simulink model "PendSwingUp"  (Simulink 8.6)
settings: Solver=ode1  SolverMode=SingleTasking  StartTime=0.0  StopTime=40  FixedStep=0.001  RelTol=1e-3
undefined symbols (not defined in the file): Advantech, PCI
libraries: sldrtlib x11, simulink x2
settings Model: Creator=pawel  LastModifiedBy=demo  SimulationMode=external  ExtModeTrigMode=oneshot  ExtModeTrigDuration=100000
settings DataIOCC: LimitDataPoints=off  SignalLoggingName=sigsOut
settings OptimizationCC: BlockReduction=off  BooleanDataType=off  InitFltsAndDblsToZero=on
settings DebuggingCC: SaveWithParameterizedLinksMsg=none  SignalResolutionControl=TryResolveAllWithWarning  SolverPrmCheckMsg=none  MultiTaskDSMMsg=warning  MultiTaskCondExecSysMsg=none  FcnCallInpInsideContextMsg=UseLocalSettings
settings HardwareCC: ProdBitPerLong=64  ProdBitPerPointer=64  ProdIntDivRoundTo=Zero  ProdEndianess=LittleEndian  ProdWordSize=64  ProdHWDeviceType=Intel->x86-64  TargetBitPerLong=64  TargetBitPerPointer=64  TargetIntDivRoundTo=Zero  TargetEndianess=LittleEndian  TargetWordSize=64  TargetHWDeviceType=Intel->x86-64
settings RTWCC: SystemTargetFile=sldrt.tlc  TemplateMakefile=sldrt.tmf  Description=Simulink Desktop Real-Time  RTWCompilerOptimization=on
settings CodeAppCC: MaxIdLength=95
settings SimulinkDesktopRealTimeCC: TargetPreCompLibLocation=C:\Program Files\MATLAB\R2015b\toolbox\sldrt\lib\win64  TargetLangStandard=C89/C90 (ANSI)  SupportVariableSizeSignals=off

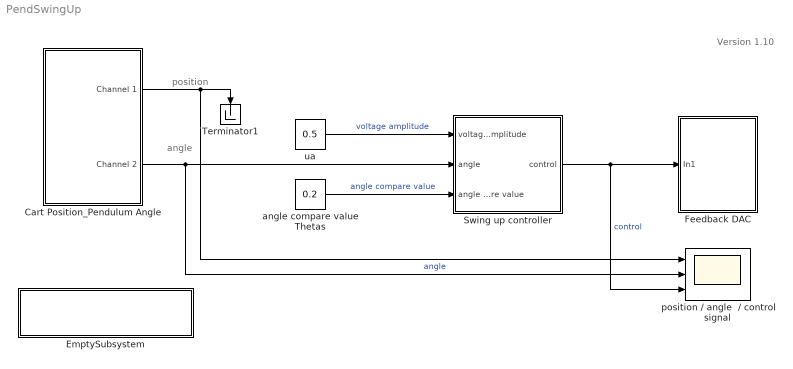
== system PendSwingUp ==
  note: position
  note: angle
  note: Version 1.10
  Cart Position_Pendulum Angle : Subsystem  mask(Feedback Encoder Block){st=0.001, of1=0, of2=-1024}
      mask prompts: st "Sample Time"; of1 "Channel 1 Offset"; of2 "Channel 2 Offset"
      mask help: Special block to use with the Feedback experiments to read encoder channels using the digital I/O lines
      mask Display:
      | image(imread('bckg.bmp'))
      | disp('PCI1711 \n Lab I/O Board \n\n\n Feedback Encoder')
  EmptySubsystem : Subsystem
      mask Display:
      | image(imread('FB-inst-blue2.jpg'))
      | disp('\n\nFeedback Instruments Limited')
  Feedback DAC : Subsystem  mask(DAC Unit for Feedback Experiments){st=0.001, ch=1}
      mask prompts: st "Sample Time"; ch "Output Channel"
      mask help:
      | Digital to Analog Output  for Feedback Experiments
      | using Advantech PCI1711  I/O board
      mask Display:
      | image(imread('bckg.bmp'))
      | disp('PCI1711 \n Lab I/O Board \n\n Feedback  DAC')
  Swing up controller : Subsystem
      mask Display:
      | image(imread('bckg.bmp'))
      | disp('Swing up \ncontroller')
  Terminator1 : Terminator
  angle compare value Thetas : Constant  Value=0.2
  position / angle  / control signal : Scope  NumInputPorts=3
      mask Display: image(imread('scope.jpg'))
  ua : Constant  Value=0.5
  wires:
  ua/1 -> Swing up controller/1(voltage amplitude)  "voltage amplitude"
  angle compare value Thetas/1 -> Swing up controller/3(angle compare value)  "angle compare value"
  Swing up controller/1(control) -> Feedback DAC/1(In1), position / angle  / control signal/3  "control"
  Cart Position_Pendulum Angle/1(Channel 1) -> Terminator1/1, position / angle  / control signal/1
  Cart Position_Pendulum Angle/2(Channel 2) -> Swing up controller/2(angle), position / angle  / control signal/2  "angle"

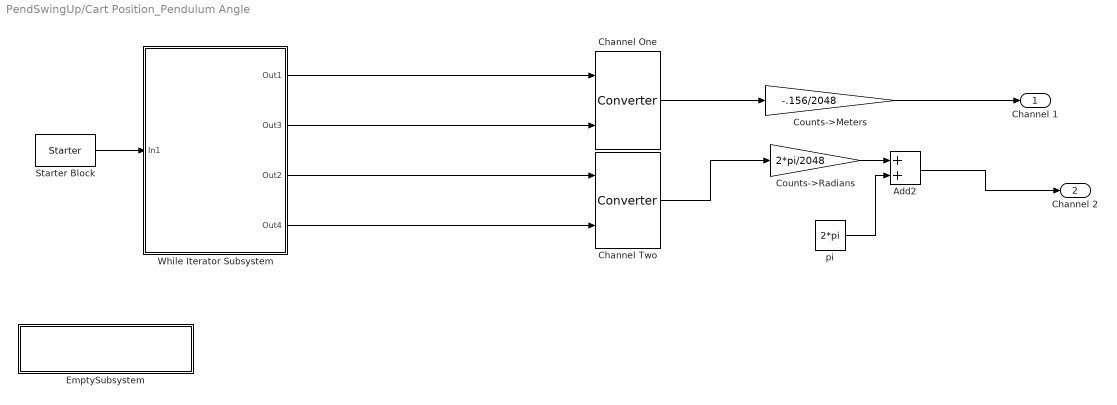
== system PendSwingUp/Cart Position_Pendulum Angle ==
  Add2 : Sum
  Channel One : S-Function  FunctionName=Converter  Parameters=of1,st  SFunctionDeploymentMode=off  EnableBusSupport=off
  Channel Two : S-Function  FunctionName=Converter  Parameters=of2,st  SFunctionDeploymentMode=off  EnableBusSupport=off
  Counts->Meters : Gain  Gain=-.156/2048  SaturateOnIntegerOverflow=on  OutDataTypeStr=Inherit: Same as input  ParamDataTypeStr=Inherit: Same as input
  Counts->Radians : Gain  Gain=2*pi/2048  SaturateOnIntegerOverflow=on  OutDataTypeStr=Inherit: Same as input  ParamDataTypeStr=Inherit: Same as input
  EmptySubsystem : Subsystem
      mask Display:
      | image(imread('FB-inst-blue2.jpg'))
      | disp('\n\nFeedback Instruments Limited')
  Starter Block : S-Function  FunctionName=Starter  Parameters=sample_time  SFunctionDeploymentMode=off  EnableBusSupport=off  mask{sample_time=st}
      mask prompts: sample_time "Sample Time:"
  While Iterator Subsystem : Subsystem  TreatAsAtomicUnit=on
  pi : Constant  Value=2*pi
  Channel 1 : Outport
  Channel 2 : Outport  Port=2
  wires:
  Add2/1 -> Channel 2/1
  Channel Two/1 -> Counts->Radians/1
  pi/1 -> Add2/2
  Counts->Radians/1 -> Add2/1
  Counts->Meters/1 -> Channel 1/1
  Starter Block/1 -> While Iterator Subsystem/1(In1)
  While Iterator Subsystem/1(Out1) -> Channel One/1
  While Iterator Subsystem/2(Out3) -> Channel One/2
  While Iterator Subsystem/3(Out2) -> Channel Two/1
  While Iterator Subsystem/4(Out4) -> Channel Two/2
  Channel One/1 -> Counts->Meters/1

== system PendSwingUp/EmptySubsystem ==

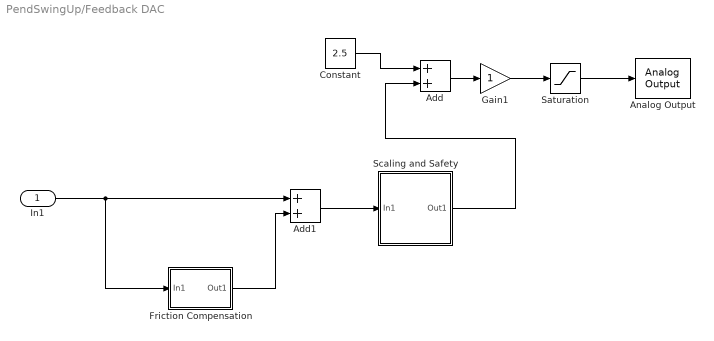
== system PendSwingUp/Feedback DAC ==
  In1 : Inport
  Add : Sum  OutDataTypeStr=Inherit: Same as first input
  Add1 : Sum
  Analog Output : sldrtlib/Analog Output  SampleTime=st  MaxMissedTicks=10  ShowMissedTicks=off  YieldWhenWaiting=off  DrvName=Advantech/PCI-1711  DrvAddress=4294967295  DrvOptions=zeros(1,0)  Channels=ch  RangeMode=1  VoltRange=2  InitialValue=2.5  FinalValue=2.5
      settings: AttributesFormatString=Advantech\nPCI-1711 [auto]
  Constant : Constant  Value=2.5
  Friction Compensation : Subsystem  mask(linear){frictionCompNeg=.1, frictionCompPos=.1}
      mask prompts: frictionCompNeg "Friction Compensation Magnitude in Negative Direction"; frictionCompPos "Friction Compensation Magnitude in Positive Direction"
      mask Display: plot(0,0,100,100,[40,30,20],[87,85,80],[46,54,54,46,46],[90,90,80,80,90],[46,45,45,46,54,55,55,54,46],[78,80,90,91,91,90,80,78,78],[51,51,49,49],[78,10,10,78],[90,80,70,60],[70,80,85,88],[20,10],[80,70],[20,20,15],[73,80,80],[85,80,80],[80,80,74])
  Gain1 : Gain
  Saturation : Saturate  UpperLimit=5.0  LowerLimit=0
  Scaling and Safety : Subsystem
  wires:
  Add1/1 -> Scaling and Safety/1(In1)
  In1/1 -> Add1/1, Friction Compensation/1(In1)
  Friction Compensation/1(Out1) -> Add1/2
  Constant/1 -> Add/1
  Saturation/1 -> Analog Output/1
  Add/1 -> Gain1/1
  Gain1/1 -> Saturation/1
  Scaling and Safety/1(Out1) -> Add/2

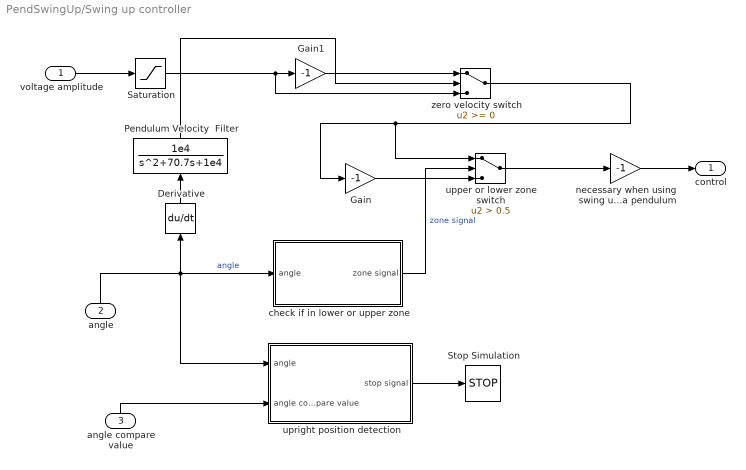
== system PendSwingUp/Swing up controller ==
  voltage amplitude : Inport
  angle : Inport  Port=2
  angle compare value : Inport  Port=3
  Derivative : Derivative
  Gain : Gain  Gain=-1
  Gain1 : Gain  Gain=-1
  Pendulum Velocity  Filter : TransferFcn  Numerator=[1e4]  Denominator=[1 70.7 1e4]
  Saturation : Saturate  UpperLimit=1  LowerLimit=0.01
  Stop Simulation : Stop
  check if in lower or upper zone : Subsystem
      mask Display:
      | image(imread('bckg.bmp'))
      | disp('lower / upper zone')
  necessary when using  swing up on a pendulum : Gain  Gain=-1
  upper or lower zone switch : Switch  Criteria=u2 > Threshold  Threshold=0.5
  upright position detection : Subsystem
      mask Display:
      | image(imread('bckg.bmp'))
      | disp('Upright position \ndetection')
  zero velocity switch : Switch
  control : Outport
  wires:
  angle compare value/1 -> upright position detection/2(angle compare value)
  angle/1 -> upright position detection/1(angle), check if in lower or upper zone/1(angle), Derivative/1  "angle"
  upright position detection/1(stop signal) -> Stop Simulation/1
  upper or lower zone switch/1 -> necessary when using  swing up on a pendulum/1
  zero velocity switch/1 -> upper or lower zone switch/1, Gain/1
  Gain1/1 -> zero velocity switch/1
  voltage amplitude/1 -> Saturation/1
  Gain/1 -> upper or lower zone switch/3
  check if in lower or upper zone/1(zone signal) -> upper or lower zone switch/2  "zone signal"
  Derivative/1 -> Pendulum Velocity  Filter/1
  Pendulum Velocity  Filter/1 -> zero velocity switch/2
  necessary when using  swing up on a pendulum/1 -> control/1
  Saturation/1 -> Gain1/1, zero velocity switch/3

== system PendSwingUp/Cart Position_Pendulum Angle/EmptySubsystem ==

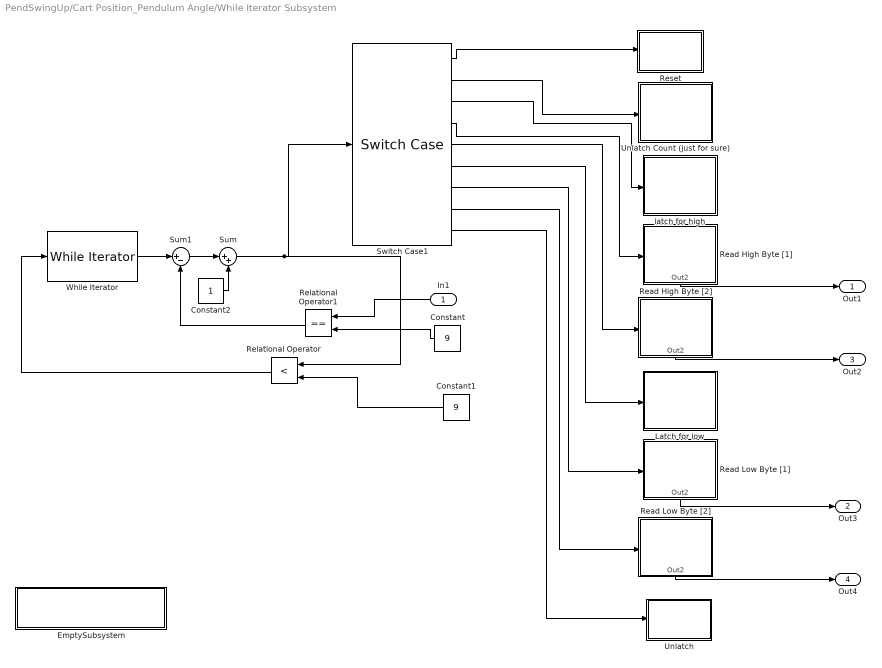
== system PendSwingUp/Cart Position_Pendulum Angle/While Iterator Subsystem ==
  In1 : Inport
  Constant : Constant  Value=9
  Constant1 : Constant  Value=9
  Constant2 : Constant
  EmptySubsystem : Subsystem
      mask Display:
      | image(imread('FB-inst-blue2.jpg'))
      | disp('\n\nFeedback Instruments Limited')
  Latch for low : Subsystem  TreatAsAtomicUnit=on
  Read High Byte [1] : Subsystem  TreatAsAtomicUnit=on
  Read High Byte [2] : Subsystem  TreatAsAtomicUnit=on
  Read Low Byte [1] : Subsystem  TreatAsAtomicUnit=on
  Read Low Byte [2] : Subsystem  TreatAsAtomicUnit=on
  Relational Operator : RelationalOperator  Operator=<  OutDataTypeStr=boolean
  Relational Operator1 : RelationalOperator  Operator===  OutDataTypeStr=boolean
  Reset : Subsystem  TreatAsAtomicUnit=on
  Sum : Sum  Inputs=|++
  Sum1 : Sum  Inputs=|+-  OutDataTypeStr=Inherit: Same as first input
  Switch Case1 : SwitchCase  CaseConditions={1,2,3,4,5,6,7,8,9}  ShowDefaultCase=off
  Unlatch : Subsystem  TreatAsAtomicUnit=on
  "Unlatch Count (just for sure) " : Subsystem  TreatAsAtomicUnit=on
  While Iterator : WhileIterator  MaxIters=9  WhileBlockType=do-while  ResetStates=reset  ShowIterationPort=on  OutputDataType=int8
  latch for high : Subsystem  TreatAsAtomicUnit=on
  Out1 : Outport
  Out3 : Outport  Port=2
  Out2 : Outport  Port=3
  Out4 : Outport  Port=4
  wires:
  Relational Operator/1 -> While Iterator/1
  In1/1 -> Relational Operator1/1
  Constant/1 -> Relational Operator1/2
  Relational Operator1/1 -> Sum1/2
  While Iterator/1 -> Sum1/1
  Switch Case1/1 -> Reset/Action
  Switch Case1/2 -> "Unlatch Count (just for sure) "/Action
  Constant1/1 -> Relational Operator/2
  Read High Byte [1]/1(Out2) -> Out1/1
  Read High Byte [2]/1(Out2) -> Out2/1
  Read Low Byte [1]/1(Out2) -> Out3/1
  Read Low Byte [2]/1(Out2) -> Out4/1
  Sum1/1 -> Sum/1
  Sum/1 -> Switch Case1/1, Relational Operator/1
  Constant2/1 -> Sum/2
  Switch Case1/3 -> latch for high/Action
  Switch Case1/4 -> Read High Byte [1]/Action
  Switch Case1/5 -> Read High Byte [2]/Action
  Switch Case1/6 -> Latch for low/Action
  Switch Case1/7 -> Read Low Byte [1]/Action
  Switch Case1/8 -> Read Low Byte [2]/Action
  Switch Case1/9 -> Unlatch/Action

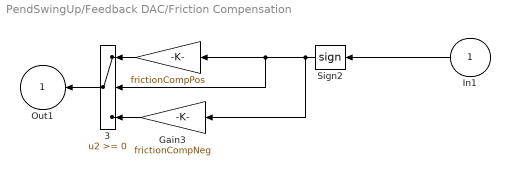
== system PendSwingUp/Feedback DAC/Friction Compensation ==
  In1 : Inport
  " " : Gain  Gain=frictionCompPos  SaturateOnIntegerOverflow=on  OutDataTypeStr=Inherit: Same as input  ParamDataTypeStr=Inherit: Same as input
  3 : Switch  SaturateOnIntegerOverflow=on  InputSameDT=on
  Gain3 : Gain  Gain=frictionCompNeg  SaturateOnIntegerOverflow=on  OutDataTypeStr=Inherit: Same as input  ParamDataTypeStr=Inherit: Same as input
  Sign2 : Signum  Tag=T
  Out1 : Outport  InitialOutput=0
  wires:
  3/1 -> Out1/1
  Sign2/1 -> 3/2, " "/1, Gain3/1
  Gain3/1 -> 3/3
  " "/1 -> 3/1
  In1/1 -> Sign2/1

== system PendSwingUp/Feedback DAC/Scaling and Safety ==
  In1 : Inport
  -1 : Gain  Gain=-1  SaturateOnIntegerOverflow=on  OutDataTypeStr=Inherit: Same as input  ParamDataTypeStr=Inherit: Same as input
  Saturation : Saturate  UpperLimit=2.5  LowerLimit=-2.5
  Out1 : Outport
  wires:
  -1/1 -> Saturation/1  "actual LoadPosition"
  In1/1 -> -1/1
  Saturation/1 -> Out1/1

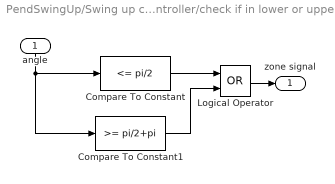
== system PendSwingUp/Swing up controller/check if in lower or upper zone ==
  angle : Inport
  Compare To Constant : simulink/Logic and Bit Operations/Compare To Constant  relop=<=  const=pi/2  OutDataTypeStr=uint8  ZeroCross=off
  Compare To Constant1 : simulink/Logic and Bit Operations/Compare To Constant  relop=>=  const=pi/2+pi  OutDataTypeStr=uint8  ZeroCross=off
  Logical Operator : Logic  Operator=OR  AllPortsSameDT=off  OutDataTypeStr=boolean
  zone signal : Outport
  wires:
  Logical Operator/1 -> zone signal/1
  angle/1 -> Compare To Constant1/1, Compare To Constant/1
  Compare To Constant1/1 -> Logical Operator/2
  Compare To Constant/1 -> Logical Operator/1

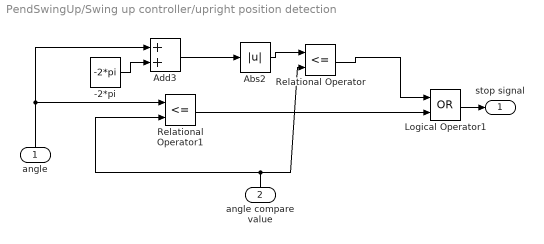
== system PendSwingUp/Swing up controller/upright position detection ==
  angle : Inport
  angle compare value : Inport  Port=2
  -2*pi : Constant  Value=-2*pi
  Abs2 : Abs
  Add3 : Sum
  Logical Operator1 : Logic  Operator=OR  AllPortsSameDT=off  OutDataTypeStr=boolean
  Relational Operator : RelationalOperator  Operator=<=  OutDataTypeStr=boolean
  Relational Operator1 : RelationalOperator  Operator=<=  OutDataTypeStr=boolean
  stop signal : Outport
  wires:
  angle compare value/1 -> Relational Operator1/2, Relational Operator/2
  Logical Operator1/1 -> stop signal/1
  angle/1 -> Relational Operator1/1, Add3/1
  Abs2/1 -> Relational Operator/1
  Add3/1 -> Abs2/1
  Relational Operator/1 -> Logical Operator1/1
  -2*pi/1 -> Add3/2
  Relational Operator1/1 -> Logical Operator1/2

== system PendSwingUp/Cart Position_Pendulum Angle/While Iterator Subsystem/EmptySubsystem ==

== system PendSwingUp/Cart Position_Pendulum Angle/While Iterator Subsystem/Latch for low ==
  Action Port : ActionPort  ActionType=case
  Constant : Constant  Value=6  OutDataTypeStr=double
  Digital Output : sldrtlib/Digital Output  SampleTime=-1  MaxMissedTicks=10  ShowMissedTicks=off  YieldWhenWaiting=off  DrvName=Advantech/PCI-1711  DrvAddress=4294967295  DrvOptions=zeros(1,0)  Channels=1  BitMode=2  InitialValue=0  FinalValue=0
      settings: AttributesFormatString=Advantech\nPCI-1711 [auto]
  wires:
  Constant/1 -> Digital Output/1

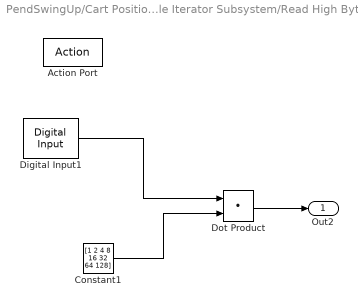
== system PendSwingUp/Cart Position_Pendulum Angle/While Iterator Subsystem/Read High Byte [1] ==
  Action Port : ActionPort  ActionType=case
  Constant1 : Constant  Value=[1 2 4 8 16 32 64 128]
  Digital Input1 : sldrtlib/Digital Input  SampleTime=-1  MaxMissedTicks=10  ShowMissedTicks=off  YieldWhenWaiting=off  DrvName=Advantech/PCI-1711  DrvAddress=4294967295  DrvOptions=zeros(1,0)  Channels=[1,2,3,4,5,6,7,8]  BitMode=1  DataType=1
      settings: AttributesFormatString=Advantech\nPCI-1711 [auto]
  Dot Product : DotProduct  InputSameDT=on  OutDataTypeStr=Inherit: Inherit via internal rule
  Out2 : Outport
  wires:
  Dot Product/1 -> Out2/1
  Constant1/1 -> Dot Product/2
  Digital Input1/1 -> Dot Product/1

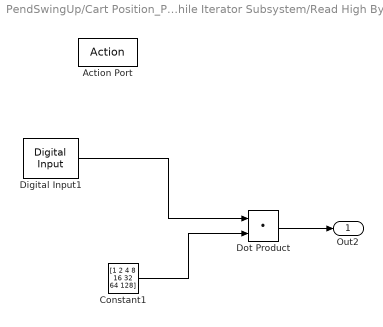
== system PendSwingUp/Cart Position_Pendulum Angle/While Iterator Subsystem/Read High Byte [2] ==
  Action Port : ActionPort  ActionType=case
  Constant1 : Constant  Value=[1 2 4 8 16 32 64 128]
  Digital Input1 : sldrtlib/Digital Input  SampleTime=-1  MaxMissedTicks=10  ShowMissedTicks=off  YieldWhenWaiting=off  DrvName=Advantech/PCI-1711  DrvAddress=4294967295  DrvOptions=zeros(1,0)  Channels=[9:16]  BitMode=1  DataType=1
      settings: AttributesFormatString=Advantech\nPCI-1711 [auto]
  Dot Product : DotProduct  InputSameDT=on  OutDataTypeStr=Inherit: Inherit via internal rule
  Out2 : Outport
  wires:
  Digital Input1/1 -> Dot Product/1
  Constant1/1 -> Dot Product/2
  Dot Product/1 -> Out2/1

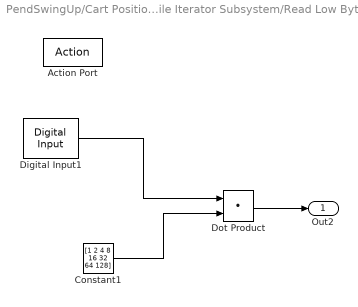
== system PendSwingUp/Cart Position_Pendulum Angle/While Iterator Subsystem/Read Low Byte [1] ==
  Action Port : ActionPort  ActionType=case
  Constant1 : Constant  Value=[1 2 4 8 16 32 64 128]
  Digital Input1 : sldrtlib/Digital Input  SampleTime=-1  MaxMissedTicks=10  ShowMissedTicks=off  YieldWhenWaiting=off  DrvName=Advantech/PCI-1711  DrvAddress=4294967295  DrvOptions=zeros(1,0)  Channels=[1:8]  BitMode=1  DataType=1
      settings: AttributesFormatString=Advantech\nPCI-1711 [auto]
  Dot Product : DotProduct  InputSameDT=on  OutDataTypeStr=Inherit: Inherit via internal rule
  Out2 : Outport
  wires:
  Digital Input1/1 -> Dot Product/1
  Constant1/1 -> Dot Product/2
  Dot Product/1 -> Out2/1

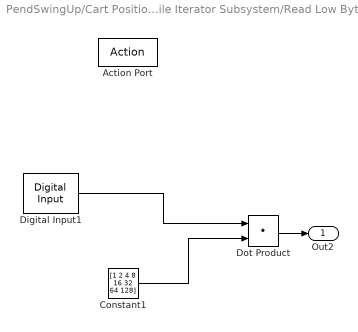
== system PendSwingUp/Cart Position_Pendulum Angle/While Iterator Subsystem/Read Low Byte [2] ==
  Action Port : ActionPort  ActionType=case
  Constant1 : Constant  Value=[1 2 4 8 16 32 64 128]
  Digital Input1 : sldrtlib/Digital Input  SampleTime=-1  MaxMissedTicks=10  ShowMissedTicks=off  YieldWhenWaiting=off  DrvName=Advantech/PCI-1711  DrvAddress=4294967295  DrvOptions=zeros(1,0)  Channels=[9:16]  BitMode=1  DataType=1
      settings: AttributesFormatString=Advantech\nPCI-1711 [auto]
  Dot Product : DotProduct  InputSameDT=on  OutDataTypeStr=Inherit: Inherit via internal rule
  Out2 : Outport
  wires:
  Constant1/1 -> Dot Product/2
  Digital Input1/1 -> Dot Product/1
  Dot Product/1 -> Out2/1

== system PendSwingUp/Cart Position_Pendulum Angle/While Iterator Subsystem/Reset ==
  Action Port : ActionPort  ActionType=case
  Constant : Constant  Value=3  OutDataTypeStr=double
  Digital Output1 : sldrtlib/Digital Output  SampleTime=-1  MaxMissedTicks=10  ShowMissedTicks=off  YieldWhenWaiting=off  DrvName=Advantech/PCI-1711  DrvAddress=4294967295  DrvOptions=zeros(1,0)  Channels=1  BitMode=2  InitialValue=0  FinalValue=0
      settings: AttributesFormatString=Advantech\nPCI-1711 [auto]
  Subsystem : Subsystem
  wires:
  Constant/1 -> Subsystem/1(In1)
  Subsystem/1(Out1) -> Digital Output1/1

== system PendSwingUp/Cart Position_Pendulum Angle/While Iterator Subsystem/Unlatch ==
  Action Port : ActionPort  ActionType=case
  Constant : Constant  Value=7  OutDataTypeStr=double
  Digital Output1 : sldrtlib/Digital Output  SampleTime=-1  MaxMissedTicks=10  ShowMissedTicks=off  YieldWhenWaiting=off  DrvName=Advantech/PCI-1711  DrvAddress=4294967295  DrvOptions=zeros(1,0)  Channels=1  BitMode=2  InitialValue=0  FinalValue=0
      settings: AttributesFormatString=Advantech\nPCI-1711 [auto]
  wires:
  Constant/1 -> Digital Output1/1

== system PendSwingUp/Cart Position_Pendulum Angle/While Iterator Subsystem/Unlatch Count (just for sure)  ==
  Action Port : ActionPort  ActionType=case
  Constant : Constant  Value=7  OutDataTypeStr=double
  Digital Output : sldrtlib/Digital Output  SampleTime=-1  MaxMissedTicks=10  ShowMissedTicks=off  YieldWhenWaiting=off  DrvName=Advantech/PCI-1711  DrvAddress=4294967295  DrvOptions=zeros(1,0)  Channels=1  BitMode=2  InitialValue=0  FinalValue=0
      settings: AttributesFormatString=Advantech\nPCI-1711 [auto]
  wires:
  Constant/1 -> Digital Output/1

== system PendSwingUp/Cart Position_Pendulum Angle/While Iterator Subsystem/latch for high ==
  Action Port : ActionPort  ActionType=case
  Constant : Constant  Value=4  OutDataTypeStr=double
  Digital Output : sldrtlib/Digital Output  SampleTime=-1  MaxMissedTicks=10  ShowMissedTicks=off  YieldWhenWaiting=off  DrvName=Advantech/PCI-1711  DrvAddress=4294967295  DrvOptions=zeros(1,0)  Channels=1  BitMode=2  InitialValue=0  FinalValue=0
      settings: AttributesFormatString=Advantech\nPCI-1711 [auto]
  wires:
  Constant/1 -> Digital Output/1

== system PendSwingUp/Cart Position_Pendulum Angle/While Iterator Subsystem/Reset/Subsystem ==
  In1 : Inport
  Constant1 : Constant  Value=7  OutDataTypeStr=double
  Digital Output : sldrtlib/Digital Output  SampleTime=-1  MaxMissedTicks=10  ShowMissedTicks=off  YieldWhenWaiting=off  DrvName=Advantech/PCI-1711  DrvAddress=4294967295  DrvOptions=zeros(1,0)  Channels=[1 2 3]  BitMode=2  InitialValue=0  FinalValue=0
      settings: AttributesFormatString=Advantech\nPCI-1711 [auto]
  Out1 : Outport
  wires:
  Constant1/1 -> Out1/1
  In1/1 -> Digital Output/1
